simulink model "task2e"  (R2016a)
settings: Solver=VariableStepAuto  StartTime=0.0  StopTime=100.0  RelTol=1e-3
values from neighbouring files (symbols this model uses):
  a1 = 2.87    [Ass_2_ailerons.m]
  a2 = -0.65    [Ass_2_ailerons.m]
  g = 9.81    [Ass_2_ailerons.m]
  kd = (2*zeta_phi*omega_n-a1)/a2    [Ass_2_ailerons.m]
  ki = 0.85    [Ass_2_ailerons.m]
  kp = 2*sign(a2)    [Ass_2_ailerons.m]
  kp_x = 7.5    [Ass_2_ailerons.m]
  Vg = 580/3.6    (= 161.111111111)    [Ass_2_ailerons.m]
settings Model: Creator=magnusschmidt  LastModifiedBy=magnusschmidt

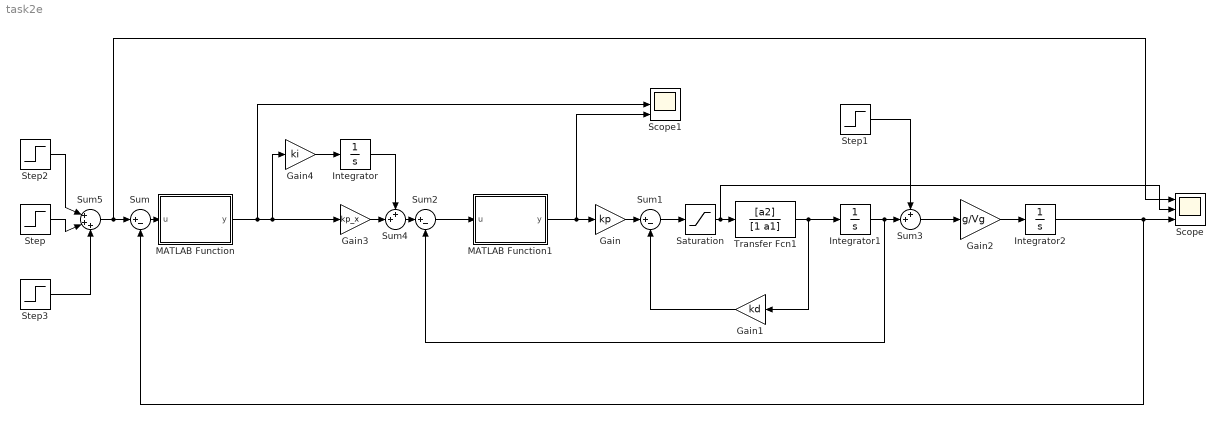
== system task2e ==
  Gain : Gain  Gain=kp
  Gain1 : Gain  Gain=kd
  Gain2 : Gain  Gain=g/Vg
  Gain3 : Gain  Gain=kp_x
  Gain4 : Gain  Gain=ki
  Integrator : Integrator
  Integrator1 : Integrator
  Integrator2 : Integrator
  MATLAB Function : MATLAB Function  TreatAsAtomicUnit=on
  MATLAB Function1 : MATLAB Function  TreatAsAtomicUnit=on
  Saturation : Saturate  UpperLimit=30  LowerLimit=-30
  Scope : Scope  NumInputPorts=3
  Scope1 : Scope  NumInputPorts=3
  Step : Step  Time=35  After=-5  SampleTime=0
  Step1 : Step  Time=0  After=1.5  SampleTime=0
  Step2 : Step  Time=10  After=5  SampleTime=0
  Step3 : Step  Time=65  After=5  SampleTime=0
  Sum : Sum  Inputs=|+-
  Sum1 : Sum  Inputs=|+-
  Sum2 : Sum  Inputs=|+-
  Sum3 : Sum  Inputs=++|
  Sum4 : Sum  Inputs=++|
  Sum5 : Sum  Inputs=|+++
  Transfer Fcn1 : TransferFcn  Numerator=[a2]  Denominator=[1 a1]
  wires:
  Transfer Fcn1/1 -> Gain1/1, Integrator1/1
  Gain1/1 -> Sum1/2
  Gain/1 -> Sum1/1
  Sum2/1 -> MATLAB Function1/1(u)
  Integrator1/1 -> Sum3/2, Sum2/2
  Sum3/1 -> Gain2/1
  Gain2/1 -> Integrator2/1
  Step1/1 -> Sum3/1
  Sum4/1 -> Sum2/1
  Gain3/1 -> Sum4/2
  Gain4/1 -> Integrator/1
  Integrator/1 -> Sum4/1
  Integrator2/1 -> Scope/3, Sum/2
  Sum5/1 -> Scope/1, Sum/1
  Step2/1 -> Sum5/1
  Step/1 -> Sum5/2
  Step3/1 -> Sum5/3
  Sum1/1 -> Saturation/1
  Saturation/1 -> Scope/2, Transfer Fcn1/1
  MATLAB Function/1(y) -> Scope1/2, Gain3/1, Gain4/1
  MATLAB Function1/1(y) -> Scope1/3, Gain/1
  Sum/1 -> MATLAB Function/1(u)

== matlab function task2e/MATLAB Function1 ==
  data: u input; y output
function y = fcn(u)

y = mod(u+180,360)-180;

== matlab function task2e/MATLAB Function ==
  data: u input; y output
function y = fcn(u)

y = mod(u+180,360)-180;
